simulink model "siasun_config_casadi_VS_lsj_sim_16a"  (R2020a)
settings: Solver=FixedStepAuto  StartTime=0.0  StopTime=20  FixedStep=0.001  RelTol=1e-3  EnableMultiTasking=on
values from neighbouring files (symbols this model uses):
  a1 = 0.040    (= 0.04)    [set_mode_parameter_siasun.m]
  a2 = 0.275    [set_mode_parameter_siasun.m]
  a3 = 0.025    [set_mode_parameter_siasun.m]
  d1 = 0.342    [set_mode_parameter_siasun.m]
  d4 = 0.280    (= 0.28)    [set_mode_parameter_siasun.m]
  fc1 = 0    [set_mode_parameter_siasun.m]
  fc2 = 0    [set_mode_parameter_siasun.m]
  fc3 = 0    [set_mode_parameter_siasun.m]
  fc4 = 0    [set_mode_parameter_siasun.m]
  fc5 = 0    [set_mode_parameter_siasun.m]
  fc6 = 0    [set_mode_parameter_siasun.m]
  fv1 = 0    [set_mode_parameter_siasun.m]
  fv2 = 0    [set_mode_parameter_siasun.m]
  fv3 = 0    [set_mode_parameter_siasun.m]
  fv4 = 0    [set_mode_parameter_siasun.m]
  fv5 = 0    [set_mode_parameter_siasun.m]
  fv6 = 0    [set_mode_parameter_siasun.m]
  Ia1 = 0    [set_mode_parameter_siasun.m]
  Ia2 = 0    [set_mode_parameter_siasun.m]
  Ia3 = 0    [set_mode_parameter_siasun.m]
  Ia4 = 0    [set_mode_parameter_siasun.m]
  Ia5 = 0    [set_mode_parameter_siasun.m]
  Ia6 = 0    [set_mode_parameter_siasun.m]
  Ic111 = 0    [set_mode_parameter_siasun.m]
  Ic112 = 0    [set_mode_parameter_siasun.m]
  Ic113 = 0    [set_mode_parameter_siasun.m]
  Ic122 = 0    [set_mode_parameter_siasun.m]
  Ic123 = 0    [set_mode_parameter_siasun.m]
  Ic133 = 1.3676    [set_mode_parameter_siasun.m]
  Ic211 = 8.8194    [set_mode_parameter_siasun.m]
  Ic212 = 0    [set_mode_parameter_siasun.m]
  Ic213 = 0    [set_mode_parameter_siasun.m]
  Ic222 = 6.0549    [set_mode_parameter_siasun.m]
  Ic223 = 0    [set_mode_parameter_siasun.m]
  Ic233 = 0.9569    [set_mode_parameter_siasun.m]
  Ic311 = 0.0332    [set_mode_parameter_siasun.m]
  Ic312 = 0    [set_mode_parameter_siasun.m]
  Ic313 = 0    [set_mode_parameter_siasun.m]
  Ic322 = 1.8442    [set_mode_parameter_siasun.m]
  Ic323 = 0    [set_mode_parameter_siasun.m]
  Ic333 = 1.0560    (= 1.056)    [set_mode_parameter_siasun.m]
  Ic411 = 0.1448    [set_mode_parameter_siasun.m]
  Ic412 = 0    [set_mode_parameter_siasun.m]
  Ic413 = 0    [set_mode_parameter_siasun.m]
  Ic422 = 0.0015    [set_mode_parameter_siasun.m]
  Ic423 = 0    [set_mode_parameter_siasun.m]
  Ic433 = 0.0822    [set_mode_parameter_siasun.m]
  Ic511 = 0    [set_mode_parameter_siasun.m]
  Ic512 = 0    [set_mode_parameter_siasun.m]
  Ic513 = 0    [set_mode_parameter_siasun.m]
  Ic522 = 0.0121    [set_mode_parameter_siasun.m]
  Ic523 = 0    [set_mode_parameter_siasun.m]
  Ic533 = 0.0299    [set_mode_parameter_siasun.m]
  Ic611 = 0.0134    [set_mode_parameter_siasun.m]
  Ic612 = 0    [set_mode_parameter_siasun.m]
  Ic613 = 0    [set_mode_parameter_siasun.m]
  Ic622 = 0    [set_mode_parameter_siasun.m]
  Ic623 = 0    [set_mode_parameter_siasun.m]
  Ic633 = 0.0051    [set_mode_parameter_siasun.m]
  m1 = 0.167    [set_mode_parameter_siasun.m]
  m2 = 1    [set_mode_parameter_siasun.m]
  m3 = 0.5    [set_mode_parameter_siasun.m]
  m4 = 0.333    [set_mode_parameter_siasun.m]
  m5 = 0.25    [set_mode_parameter_siasun.m]
  m6 = 0.2    [set_mode_parameter_siasun.m]
  mc11 = 0    [set_mode_parameter_siasun.m]
  mc12 = 0    [set_mode_parameter_siasun.m]
  mc13 = 0.2    [set_mode_parameter_siasun.m]
  mc21 = 0.1291    [set_mode_parameter_siasun.m]
  mc22 = 0    [set_mode_parameter_siasun.m]
  mc23 = 3.3117    [set_mode_parameter_siasun.m]
  mc31 = 1.6484    [set_mode_parameter_siasun.m]
  mc32 = 0    [set_mode_parameter_siasun.m]
  mc33 = 0.8748    [set_mode_parameter_siasun.m]
  mc41 = 0.3200    (= 0.32)    [set_mode_parameter_siasun.m]
  mc42 = 0.2324    [set_mode_parameter_siasun.m]
  mc43 = 0.7083    [set_mode_parameter_siasun.m]
  mc51 = 0.4574    [set_mode_parameter_siasun.m]
  mc52 = 0    [set_mode_parameter_siasun.m]
  mc53 = 0.6427    [set_mode_parameter_siasun.m]
  mc61 = 0.3200    (= 0.32)    [set_mode_parameter_siasun.m]
  mc62 = -0.0513    [set_mode_parameter_siasun.m]
  mc63 = 0.6417    [set_mode_parameter_siasun.m]
undefined symbols (not defined in the file or in its folder): X, Y, Z
libraries: sm_lib x224, nesl_utility x124, simulink x8
(part 11 of 11)

== matlab function siasun_config_casadi_VS_lsj_sim_16a/siasun_rel/Robot/Robot/robot/friction ==
  data: u input; y output; fv input; fc input
function y = fcn(u,fv,fc)
%#codegen


% fv1=100; fc1=80; fv2=150; fc2=100; fv3=100; fc3=50; fv4=80; fc4=80; fv5=50; fc5=30; fv6=30; fc6=10;
fv1=fv(1); fc1=fc(1); fv2=fv(2); fc2=fc(2); fv3=fv(3); fc3=fc(3); fv4=fv(4); fc4=fc(4); fv5=fv(5); fc5=fc(5); fv6=fv(6); fc6=fc(6);
y=[0;0;0;0;0;0];
y(1)=(fv1*u(1)+fc1*sign(u(1)));
y(2)=(fv2*u(2)+fc2*sign(u(2)));
y(3)=(fv3*u(3)+fc3*sign(u(3)));
y(4)=(fv4*u(4)+fc4*sign(u(4)));
y(5)=(fv5*u(5)+fc5*sign(u(5)));
y(6)=(fv6*u(6)+fc6*sign(u(6)));

end

== matlab function siasun_config_casadi_VS_lsj_sim_16a/siasun_obs/Robot/Robot/robot/Jm ==
  data: u input; y output; Jm input
function y = fcn(u,Jm)
%#codegen

% Jm=[200; 250; 150; 100; 50; 20];%关节惯性
y = Jm.*u;
end

== matlab function siasun_config_casadi_VS_lsj_sim_16a/siasun_obs/Robot/Robot/robot/friction ==
  data: u input; y output; fv input; fc input
function y = fcn(u,fv,fc)
%#codegen


% fv1=100; fc1=80; fv2=150; fc2=100; fv3=100; fc3=50; fv4=80; fc4=80; fv5=50; fc5=30; fv6=30; fc6=10;
fv1=fv(1); fc1=fc(1); fv2=fv(2); fc2=fc(2); fv3=fv(3); fc3=fc(3); fv4=fv(4); fc4=fc(4); fv5=fv(5); fc5=fc(5); fv6=fv(6); fc6=fc(6);
y=[0;0;0;0;0;0];
y(1)=(fv1*u(1)+fc1*sign(u(1)));
y(2)=(fv2*u(2)+fc2*sign(u(2)));
y(3)=(fv3*u(3)+fc3*sign(u(3)));
y(4)=(fv4*u(4)+fc4*sign(u(4)));
y(5)=(fv5*u(5)+fc5*sign(u(5)));
y(6)=(fv6*u(6)+fc6*sign(u(6)));

end

== matlab function siasun_config_casadi_VS_lsj_sim_16a/DH-CC1 ==
  data: KPS44 input; KPS6 output
function KPS6  = FK(KPS44)
%% parameter
rpy = zeros(1,3);
eps = 0.000001;
%% input 
T=[1 0 0 0;0 1 0 0; 0 0 1 0];
G=KPS44;
H =T * ( G * [0;0;0;1]);
%%
rpy(2) = atan2(-KPS44(3,1),sqrt(KPS44(1,1)*KPS44(1,1)+KPS44(2,1)*KPS44(2,1)));
if (abs(abs(rpy(2)) - pi / 2.0) < eps)
	if (rpy(2) > 0) 
        rpy(2) = pi / 2.0;
        rpy(3) = 0.0;
        rpy(1) = atan2(KPS44(1,2),KPS44(2,2));
    else
    rpy(2) = -pi / 2.0;
	rpy(3) = 0.0;
	rpy(1) = -atan2(KPS44(1,2), KPS44(2,2));
	end
else
	cp = cos(rpy(2));
	rpy(3) = atan2(KPS44(2,1)/cp,KPS44(1,1)/cp);
	rpy(1) = atan2(KPS44(3,2)/cp, KPS44(3,3)/cp);
end
KPS6 = [H' rpy]; 
end

== matlab function siasun_config_casadi_VS_lsj_sim_16a/DH1 ==
  data: Radian input; KPS44 output
function KPS44  = FK(Radian)

%% input 
theta1 = Radian(1);
theta2 = Radian(2);
theta3 = Radian(3);
theta4 = Radian(4);
theta5 = Radian(5);
theta6 = Radian(6);
offset2 = -pi/2; offset3 =0;
Q=[theta1;theta2+offset2;theta3+offset3;theta4;theta5;theta6];
%% D-H parameters 
%XB4
% d1=342;a1=40;a2=275;a3=25;d4=280;dt=73;d3=0;

%siasun
d1=330;a1=40;a2=315;a3=70;d4=324.5;dt=78;d3=0;

%XB7
% d1=380;a1=30;a2=340;a3=35;d4=345;dt=87;d3=0;

Tbase = [1 0 0 0;
        0 1 0 0;
        0 0 1 d1;
        0 0 0 1];
Ttool = [1 0 0 0;
        0 1 0 0;
        0 0 1 dt;
        0 0 0 1];
%% output
II = zeros(4,4);

%% T1~T6
s1=sin(Q(1));s2=sin(Q(2));s3=sin(Q(3));s4=sin(Q(4));s5=sin(Q(5));s6=sin(Q(6));
c1=cos(Q(1));c2=cos(Q(2));c3=cos(Q(3));c4=cos(Q(4));c5=cos(Q(5));c6=cos(Q(6));

t14 = a1*c1 + a3*(c1*c2*c3 - c1*s2*s3) - d3*s1 - d4*(c1*c2*s3 + c1*c3*s2) + a2*c1*c2;
t24 = a1*s1 + c1*d3 + a3*(c2*c3*s1 - s1*s2*s3) - d4*(c2*s1*s3 + c3*s1*s2) + a2*c2*s1;
t34 =-a2*s2 - a3*(c2*s3 + c3*s2) - d4*(c2*c3 - s2*s3);

t11 =s6*(c4*s1 - s4*(c1*c2*c3 - c1*s2*s3)) - c6*(s5*(c1*c2*s3 + c1*c3*s2) - c5*(s1*s4 + c4*(c1*c2*c3 - c1*s2*s3)));
t21 = - c6*(s5*(c2*s1*s3 + c3*s1*s2) + c5*(c1*s4 - c4*(c2*c3*s1 - s1*s2*s3))) - s6*(c1*c4 + s4*(c2*c3*s1 - s1*s2*s3));
t31 = s4*s6*(c2*s3 + c3*s2) - c6*(s5*(c2*c3 - s2*s3) + c4*c5*(c2*s3 + c3*s2));
t12 = s6*(s5*(c1*c2*s3 + c1*c3*s2) - c5*(s1*s4 + c4*(c1*c2*c3 - c1*s2*s3))) + c6*(c4*s1 - s4*(c1*c2*c3 - c1*s2*s3));
t22 =s6*(s5*(c2*s1*s3 + c3*s1*s2) + c5*(c1*s4 - c4*(c2*c3*s1 - s1*s2*s3))) - c6*(c1*c4 + s4*(c2*c3*s1 - s1*s2*s3));
t32 =s6*(s5*(c2*c3 - s2*s3) + c4*c5*(c2*s3 + c3*s2)) + c6*s4*(c2*s3 + c3*s2);
t13= - c5*(c1*c2*s3 + c1*c3*s2) - s5*(s1*s4 + c4*(c1*c2*c3 - c1*s2*s3));
t23 = s5*(c1*s4 - c4*(c2*c3*s1 - s1*s2*s3)) - c5*(c2*s1*s3 + c3*s1*s2);
t33 = c4*s5*(c2*s3 + c3*s2) - c5*(c2*c3 - s2*s3);


II = [t11 t12 t13 t14;
         t21 t22 t23 t24;
         t31 t32 t33 t34;
         0 0 0 1];
     
KPS44 = Tbase*II*Ttool;

end

== matlab function siasun_config_casadi_VS_lsj_sim_16a/xb4_obs/Robot/Robot/robot/Jm ==
  data: u input; y output; Jm input
function y = fcn(u,Jm)
%#codegen

% Jm=[200; 250; 150; 100; 50; 20];%关节惯性
y = Jm.*u;
end
